simulink model "boostObserver_original"  (R2020a)
settings: Solver=ode45  StartTime=0.0  StopTime=1  FixedStep=0.0005  AbsTol=1e-06  EnableMultiTasking=on
InitFcn:
  | kp=0.01;
  | ki=0.01;
  | 
  | k=2;
  | em=100000000;
  | GE=1/em;
  | GU=k*ki/GE;
  | GCE=k*kp/GU;
model workspace (MAT data in the model file):
  time = 0.8
values from neighbouring files (symbols this model uses):
  A1 = obj.boostConverter.A1    [BoostController.m]    (also in BoostConverter.m = [-obj.R/obj.L 0;0 -1/(obj.Ro*obj.C)]; BuckBoostConverter.m = [-obj.R/obj.L 0;0 -1/(obj.Ro*obj.C)]; obsmc.m = Asigma{1,1}; workspace_atual.mat = [-16.4  0; 0  -3.50877192982])
  A1aug = [-16.4  0  0; 0  -3.50877192982  0; 0  1  0]    [workspace_atual.mat]    (also in workspace_certo.mat)
  A2 = obj.boostConverter.A2    [BoostController.m]    (also in BoostConverter.m = [-obj.R/obj.L -1/obj.L;1/obj.C -1/(obj.Ro*obj.C)]; BuckBoostConverter.m = [-obj.R/obj.L 1/obj.L;-1/obj.C -1/(obj.Ro*obj.C)]; obsmc.m = Asigma{1,2}; workspace_atual.mat = [-16.4  -200; 350.877192982  -3.50877192982])
  B1 = obj.boostConverter.B1    [BoostController.m]    (also in BoostConverter.m = [1/obj.L;0]; BuckBoostConverter.m = [1/obj.L;0]; obsmc.m = Bsigma{1,1}; workspace_atual.mat = [200 0])
  B2aug = [200 0 -2]    [workspace_atual.mat]    (also in workspace_certo.mat)
  c = 0.00285    [workspace_atual.mat]    (also in workspace_certo.mat)
  CiL = [0 1]    [workspace_atual.mat]    (also in workspace_certo.mat)
  Cmatrix = [1  0; 0  1]    [workspace_atual.mat]    (also in workspace_certo.mat)
  CVc = [1 0]    [workspace_atual.mat]    (also in workspace_certo.mat)
  deltaA = [0  200  0; -350.877192982  0  0; 0  0  0]    [workspace_atual.mat]    (also in workspace_certo.mat)
  FaultClass = 0    [BoostFaultSimulation.m]    (also in workspace_atual.mat = 1; workspace_certo.mat = 1)
  ie = equilibriumcurrent(obj,ve)    [BoostConverter.m]    (also in BoostFaultSimulation.m = 7.6251; BuckBoostConverter.m = i_e(obj,ve); workspace_atual.mat = 7.6251; workspace_certo.mat = 7.6251)
  iLFaultSwitch = 0    [BoostFaultSimulation.m]    (also in workspace_atual.mat; workspace_certo.mat)
  iLFaultTime = 1.70    (= 1.7)    [BoostFaultSimulation.m]    (also in workspace_atual.mat; workspace_certo.mat)
  Kg = [-8 -0.8 -2.3]    [workspace_atual.mat]    (also in workspace_certo.mat)
  Lnew1 = [0.000426144297292  -1.37628182296; -0.636691353583  10000.3869597]    [workspace_atual.mat]    (also in workspace_certo.mat = [0.00144628510103  0.00148492117427; 0.000288596381821  0.00)
  Lnew2 = [0.000454345330516  -0.588943865675; 0.999552025739  4999.94512306]    [workspace_atual.mat]    (also in workspace_certo.mat = [0.00251672143174  0.00251025627081; 6.60131109739e-05  6.53)
  LoadAddFactor = 0.30    (= 0.3)    [BoostFaultSimulation.m]    (also in workspace_atual.mat; workspace_certo.mat)
  LoadRemoveFactor = 0.30    (= 0.3)    [BoostFaultSimulation.m]    (also in workspace_atual.mat; workspace_certo.mat)
  Lobsmc = L    [obsmc.m]    (also in workspace_atual.mat = [-39.840516804 -308.588682873 -0.55787282725]; workspace_certo.mat = [-39.840516804 -308.588682873 -0.55787282725])
  R = 0.1    [boostResults2Latex.m]    (also in workspace_atual.mat = 0.082; workspace_certo.mat = 0.082)
  ReconfigSwitch = 0    [BoostFaultSimulation.m]    (also in workspace_atual.mat; workspace_certo.mat)
  ReconfigTime = 1.707    [BoostFaultSimulation.m]    (also in workspace_atual.mat; workspace_certo.mat)
  Ro = 100    [BoostFaultSimulation.m]    (also in boostResults2Latex.m = 10; workspace_atual.mat; workspace_certo.mat)
  Smep = 80    [workspace_atual.mat]    (also in workspace_certo.mat)
  SmFrequency = 7000    [workspace_atual.mat]    (also in workspace_certo.mat)
  SmiLGain = 8    [workspace_atual.mat]    (also in workspace_certo.mat)
  SmIntegralGain = 2.3    [workspace_atual.mat]    (also in workspace_certo.mat)
  SmVcGain = 0.8    [workspace_atual.mat]    (also in workspace_certo.mat)
  SourceAddFactor = 0.10    (= 0.1)    [BoostFaultSimulation.m]    (also in workspace_atual.mat; workspace_certo.mat)
  SourceAddSwitch = 0    [BoostFaultSimulation.m]    (also in workspace_atual.mat; workspace_certo.mat)
  SourceRemoveFactor = 0.10    (= 0.1)    [BoostFaultSimulation.m]    (also in workspace_atual.mat; workspace_certo.mat)
  T_1 = [1 -13715.5123667]    [workspace_atual.mat]    (also in workspace_certo.mat)
  T_2 = [-0.00750867981628 1]    [workspace_atual.mat]    (also in workspace_certo.mat)
  Ts = 0.0001    [workspace_atual.mat]    (also in workspace_certo.mat)
  ueq = 0.5    [workspace_atual.mat]    (also in workspace_certo.mat)
  VcFaultSwitch = 0    [BoostFaultSimulation.m]    (also in workspace_atual.mat; workspace_certo.mat)
  VcFaultTime = 1.70    (= 1.7)    [BoostFaultSimulation.m]    (also in workspace_atual.mat; workspace_certo.mat)
  ve = 380    [BoostFaultSimulation.m]    (also in boostResults2Latex.m = 100; workspace_atual.mat; workspace_certo.mat)
  Wobsmc = W    [obsmc.m]    (also in workspace_atual.mat = [3.6619016063  2.99523180353  1.23384935718; 2.99523180353  ; workspace_certo.mat = [3.66188539077  2.99521892267  1.23384557868; 2.99521892267 )
  x_e = [ie;ve]    [BoostConverter.m]    (also in BuckBoostConverter.m)
  xe = obj.boostConverter.equilibriumstate(ve)    [BoostController.m]    (also in workspace_atual.mat = [7.62509288104 380]; workspace_certo.mat = [7.62509288104 380])
libraries: PhdLibrary x17, neural x12, powerlib_meascontrol x3, dspstat3 x1, powerlib x1
(part 1 of 2)
settings Model: SimulationMode=accelerator  Creator=d13go  LastModifiedBy=d13go
settings SolverCC: MaxConsecutiveZCs=10000  ZeroCrossAlgorithm=Adaptive  DecoupledContinuousIntegration=on  MinimalZcImpactIntegration=on
settings DataIOCC: SaveFinalState=on  SaveState=on  LoggingToFile=on
settings OptimizationCC: DefaultParameterBehavior=Inlined  UseDivisionForNetSlopeComputation=on  GainParamInheritBuiltInType=on  UseFloatMulNetSlope=on  InlineInvariantSignals=on  EfficientFloat2IntCast=on  LifeSpan=1
settings DebuggingCC: ReadBeforeWriteMsg=DisableAll  WriteAfterWriteMsg=DisableAll  WriteAfterReadMsg=DisableAll  AlgebraicLoopMsg=error  MaxConsecutiveZCsMsg=warning  MaskedZcDiagnostic=none  IgnoredZcDiagnostic=none  MultiTaskDSMMsg=none  SFUnexpectedBacktrackingDiag=warning  SFNoUnconditionalDefaultTransitionDiag=warning  ArithmeticOperatorsInVariantConditions=warning
settings HardwareCC: ProdLongLongMode=on
settings ModelReferenceCC: UpdateModelReferenceTargets=IfOutOfDate
settings SFSimCC: SFSimEcho=off  SimUseLocalCustomCode=off  MATLABDynamicMemAlloc=off  CustomCodeUndefinedFunction=UseInterfaceOnly
settings RTWCC: GenerateReport=on  RTWUseLocalCustomCode=off  LaunchReport=on
settings CodeAppCC: ForceParamTrailComments=on
settings GRTTargetCC: TargetLangStandard=C89/C90 (ANSI)  CombineSignalStateStructs=on  MatFileLogging=off  SupportVariableSizeSignals=on
settings ConfigComp: CovMetricSettings=dw  CovHtmlReporting=on  CovSaveCumulativeToWorkspaceVar=on  CovSaveSingleToWorkspaceVar=on  CovExternalEMLEnable=off
settings SimscapeCC: SimscapeNormalizeSystem=off

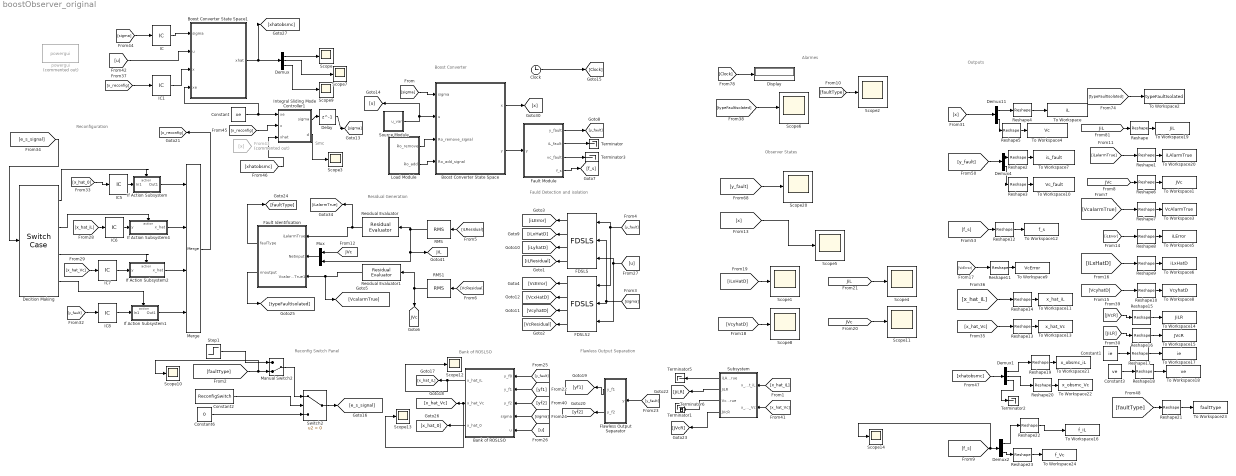
== system boostObserver_original ==
  note: Alarmes
  note: Smc
  note: Fauld Detection and isolation
  note: Outputs
  note: Bank of ROSLSO
  note: Flawless Output
      | Separation
  note: Observer States
  note: Residual Generation
  note: Reconfiguration
  note: Reconfig Switch Panel
  note: Boost Converter
  Bank of ROSLSO : Subsystem
  Boost Converter State Space : Subsystem  AncestorBlock="PhdLibrary/Boost Converter  State Space"  mask(Boots State-Space model){A1=A1, A2=A2, B1=B1, R=R, Ro=Ro, Cmatrix=Cmatrix, c=c, LoadAddFactor=LoadAddFactor, LoadRemoveFactor=LoadRemoveFactor}
      mask prompts: A1 "A1 matrix:"; A2 "A2 matrix:"; B1 "B matrix:"; R "Resistance:"; Ro "Output Resistance:"; Cmatrix "Output Matrix:"; c "Capacitance:"; LoadAddFactor "Load add factor:"; LoadRemoveFactor "Load remove factor"
      mask help: Boots State-Space model
      mask Display: disp('Boost')
  Boost Converter State Space1 : Subsystem  mask(Boots State-Space model){A1=A1, A2=A2, B1=B1, R=R, Ro=Ro, Cmatrix=Cmatrix, c=c, LoadAddFactor=LoadAddFactor, LoadRemoveFactor=LoadRemoveFactor}
      mask prompts: A1 "A1 matrix:"; A2 "A2 matrix:"; B1 "B matrix:"; R "Resistance:"; Ro "Output Resistance:"; Cmatrix "Output Matrix:"; c "Capacitance:"; LoadAddFactor "Load add factor:"; LoadRemoveFactor "Load remove factor"
      mask help: Boots State-Space model
      mask Display: disp('Boost')
  Clock : Clock
  Constant : Constant  Value=xe  VectorParams1D=off
  Constant1 : Constant  Value=ie  VectorParams1D=off
  Constant2 : Constant  Value=ReconfigSwitch
  Constant3 : Constant  Value=ve  VectorParams1D=off
  Constant6 : Constant  Value=0
  Decition Making : SwitchCase  CaseConditions={[0],[1],[2]}
  Delay : Delay  DelayLength=1
  Demux : Demux  Outputs=3
  Demux1 : Demux  Outputs=3
  Demux11 : Demux  Outputs=2
  Demux2 : Demux  Outputs=2
  Demux4 : Demux  Outputs=2
  Display : Display
  FDSLS : PhdLibrary/FDSLS  A1=A1  A2=A2  B1=B1  B2=B2  L=Lnew1  yhat0=[0;0]  x0=[0;0]  Qr=[1 0]
      settings: SourceProductName=Phd Diego
  FDSLS2 : PhdLibrary/FDSLS  A1=A1  A2=A2  B1=B1  B2=B2  L=Lnew2  yhat0=[0;0]  x0=[0;0]  Qr=[0 1]
      settings: SourceProductName=Phd Diego
  Fault Identification : Subsystem
  Fault Module : Subsystem
  Flawless Output Separator : Subsystem  mask(Flawless Output Separator){Cf1=CiL, Cf2=CVc}
      mask prompts: Cf1 "Fault matrix 1"; Cf2 "Fault matrix 2"
      mask help: Separates the 2x1 output
  From43 : From  Commented=on  GotoTag=x
  IC : InitialCondition
  IC{1,5..8} (5 alike) : InitialCondition  Value=[0;0]
  If Action Subsystem : Subsystem  TreatAsAtomicUnit=on
  If Action Subsystem1 : Subsystem  TreatAsAtomicUnit=on
  If Action Subsystem2 : Subsystem  TreatAsAtomicUnit=on
  If Action Subsystem4 : Subsystem  TreatAsAtomicUnit=on
  Integral Sliding Mode Controller1 : Subsystem  mask(Sliding mode controller){KiVc=SmIntegralGain, KVc=SmVcGain, ueq=ueq, Smep=Smep, KiL=SmiLGain, Freq=SmFrequency, x0=[0;0], Ts=0}
      mask prompts: KiVc "Integral voltage gain"; KVc "Voltage gain"; ueq "Equilibrium signal"; Smep "Surface limit layer"; KiL "Current gain"; Freq "Frequency"; x0 "Initial state:"; Ts "Sample Time"
      mask help: Sliding mode controller with integral for boost converter
  Load Module : Subsystem
  Manual Switch2 : ManualSwitch  CurrentSetting=0
  Merge : Merge  Inputs=4
  Mux : Mux  Inputs=2
  RMS : powerlib_meascontrol/Measurements/RMS  TrueRMS=on  Freq=RMSfrequency  RMSInit=0  Ts=Ts
  RMS1 : powerlib_meascontrol/Measurements/RMS  TrueRMS=on  Freq=RMSfrequency  RMSInit=0  Ts=Ts
  Reshape{,1..23} (24 alike) : Reshape
  Residual Evaluator : PhdLibrary/Residual Evaluator  Jth=iLJth
      settings: SourceProductName=Phd Diego
  Residual Evaluator1 : PhdLibrary/Residual Evaluator  Jth=VcJth
      settings: SourceProductName=Phd Diego
  Scope{,1..14,20} (16 alike) : Scope
  Source Module : Subsystem
  Step1 : Step  Time=ReconfigTime  After=FaultClass  SampleTime=0
  Subsystem : Subsystem
  Switch2 : Switch  Criteria=u2 > Threshold
  Terminator{,1..3,5..6} (6 alike) : Terminator
  To Workspace : ToWorkspace  VariableName=iL  SaveFormat=Timeseries  SampleTime=-1
  To Workspace1 : ToWorkspace  VariableName=JVc  SaveFormat=Timeseries  SampleTime=-1
  To Workspace10 : ToWorkspace  VariableName=Vc_fault  SaveFormat=Timeseries  SampleTime=-1
  To Workspace11 : ToWorkspace  VariableName=x_hat_iL  SaveFormat=Timeseries  SampleTime=-1
  To Workspace12 : ToWorkspace  VariableName=f_s  SaveFormat=Timeseries  SampleTime=-1
  To Workspace13 : ToWorkspace  VariableName=x_hat_Vc  SaveFormat=Timeseries  SampleTime=-1
  To Workspace14 : ToWorkspace  VariableName=JiLR  SaveFormat=Timeseries  SampleTime=-1
  To Workspace15 : ToWorkspace  VariableName=JVcR  SaveFormat=Timeseries  SampleTime=-1
  To Workspace16 : ToWorkspace  VariableName=f_iL  SaveFormat=Timeseries  SampleTime=-1
  To Workspace17 : ToWorkspace  VariableName=ie  SaveFormat=Timeseries  SampleTime=-1
  To Workspace18 : ToWorkspace  VariableName=ve  SaveFormat=Timeseries  SampleTime=-1
  To Workspace19 : ToWorkspace  VariableName=JiL  SaveFormat=Timeseries  SampleTime=-1
  To Workspace2 : ToWorkspace  VariableName=typeFaultIsolated  SaveFormat=Timeseries  SampleTime=-1
  To Workspace20 : ToWorkspace  VariableName=iLAlarmTrue  SaveFormat=Timeseries  SampleTime=-1
  To Workspace21 : ToWorkspace  VariableName=x_obsmc_iL  SaveFormat=Timeseries  SampleTime=-1
  To Workspace22 : ToWorkspace  VariableName=x_obsmc_Vc  SaveFormat=Timeseries  SampleTime=-1
  To Workspace23 : ToWorkspace  VariableName=faultType  SaveFormat=Timeseries  SampleTime=-1
  To Workspace24 : ToWorkspace  VariableName=f_Vc  SaveFormat=Timeseries  SampleTime=-1
  To Workspace3 : ToWorkspace  VariableName=VcAlarmTrue  SaveFormat=Timeseries  SampleTime=-1
  To Workspace4 : ToWorkspace  VariableName=Vc  SaveFormat=Timeseries  SampleTime=-1
  To Workspace5 : ToWorkspace  VariableName=iLError  SaveFormat=Timeseries  SampleTime=-1
  To Workspace6 : ToWorkspace  VariableName=iLxHatD  SaveFormat=Timeseries  SampleTime=-1
  To Workspace7 : ToWorkspace  VariableName=iL_fault  SaveFormat=Timeseries  SampleTime=-1
  To Workspace8 : ToWorkspace  VariableName=VcyhatD  SaveFormat=Timeseries  SampleTime=-1
  To Workspace9 : ToWorkspace  VariableName=VcError  SaveFormat=Timeseries  SampleTime=-1
  powergui : powerlib/powergui  Priority=1  Commented=on  SimulationMode=Discrete  SampleTime=50e-6  frequency=60  Iterations=50  frequencyindice=0  Pbase=100e6  ErrMax=1e-4  UnitsV=kV  UnitsW=MW  buscounter=0  FunctionMessages=off  echomessages=off  EnableUseOfTLC=off  CurrentSourceSwitches=off  DisableSnubberDevices=off  DisableRonSwitches=off  DisableVfSwitches=off  DisplayEquations=off  AutomaticDiscreteSolvers=off  SolverType=Tustin/Backward Euler (TBE)  Interpol=off  ExternalGateDelay=off  methode=off  Ts=100  x0status=blocks  SPID=on  SwTol=0  HookPort=off  NonlinearTolerance=1e-4  nMaxIteration=100  ContinueOnMaxIteration=off  RestoreLinks=warning  ResistiveCurrentMeasurement=off  Frange=[0:2:500]  Ylog=off  Xlog=on  ShowGrid=off  save=off  variable=ZData  structure=0  ZoomFFT=off  StartTime=0.0  cycles=1  DisplayStyle=1  fundamental=60  FreqAxis=off  MaxFrequency=1000  frequencyindicesteady=1  RmsSteady=1  display=off
  tag scope: JVc=global, JiL=global
  wires:
  Switch2/1 -> [e_s_signal]
  Reshape9/1 -> To Workspace6/1
  [y_fault] -> FDSLS2/1, FDSLS/1
  Demux4/1 -> Reshape2/1
  If Action Subsystem2/1(x_hat) -> Merge/3
  Decition Making/4 -> If Action Subsystem1/Action
  [iLResidual] -> RMS/1
  [faultType] -> Scope2/1
  [faultType] -> Scope10/1, Manual Switch2/2
  Merge/1 -> [x_reconfig]
  Clock/1 -> [Clock]
  Boost Converter State Space/1(x) -> [x]
  IC7/1 -> If Action Subsystem2/1(y)
  Fault Module/2(iL_fault) -> Terminator/1
  [JVc] -> Scope11/1
  [x_hat_Vc] -> Reshape13/1
  Demux4/2 -> Reshape3/1
  IC5/1 -> If Action Subsystem/1(In1)
  If Action Subsystem1/1(Out1) -> Merge/4
  Manual Switch2/1 -> Switch2/1
  Reshape7/1 -> To Workspace3/1
  Flawless Output Separator/2(y_f2) -> [yf2]
  Load Module/1(Ro_remove) -> Boost Converter State Space/3(Ro_remove_signal)
  [u] -> Bank of ROSLSO/5(u)
  Reshape12/1 -> To Workspace12/1
  [y_fault] -> Flawless Output Separator/1(y)
  Constant6/1 -> Switch2/3
  Reshape2/1 -> To Workspace7/1
  Fault Identification/2(nnoutput) -> [typeFaultIsolated]
  Residual Evaluator/1 -> Fault Identification/1(iLalarmTrue), [iLalarmTrue]
  Mux/1 -> Fault Identification/2(Netinput)
  Decition Making/3 -> If Action Subsystem2/Action
  Decition Making/2 -> If Action Subsystem4/Action
  [JVcR] -> Reshape15/1
  Residual Evaluator1/1 -> [VcalarmTrue], Fault Identification/3(VcalarmTrue1)
  Fault Identification/1(faulType) -> [faultType]
  [y_fault] -> Scope20/1
  [JiL] -> Scope4/1
  [VcyhatD] -> Reshape10/1
  [x] -> Demux11/1
  FDSLS2/2 -> [VcxHatD]
  Load Module/2(Ro_add) -> Boost Converter State Space/4(Ro_add_signal)
  Source Module/1(u_var) -> [u], Boost Converter State Space/2(u)
  Fault Module/4(f_s) -> [f_s]
  Boost Converter State Space/2(y) -> Fault Module/1(y)
  [VcResidual] -> RMS1/1
  [sigma] -> FDSLS2/2, FDSLS/2
  Reshape16/1 -> To Workspace15/1
  Demux11/1 -> Reshape4/1
  Bank of ROSLSO/1(x_hat_iL) -> Scope12/1, [x_hat_iL]
  Reshape13/1 -> To Workspace13/1
  RMS1/1 -> Residual Evaluator1/1, [JVc]
  RMS/1 -> [JiL], Mux/2, Residual Evaluator/1
  Reshape15/1 -> To Workspace14/1
  [iLalarmTrue] -> Reshape1/1
  Reshape1/1 -> To Workspace20/1
  Flawless Output Separator/1(y_f1) -> [yf1]
  Reshape14/1 -> To Workspace11/1
  [sigma] -> Boost Converter State Space/1(sigma)
  [VcError] -> Reshape11/1
  [x] -> Scope5/1
  FDSLS/4 -> [iLResidual]
  FDSLS2/3 -> [VcyhatD]
  [y_fault] -> Bank of ROSLSO/1(y_f0)
  Reshape4/1 -> To Workspace/1
  FDSLS2/1 -> [VcError]
  [VcyhatD] -> Scope8/1
  Reshape11/1 -> To Workspace9/1
  [y_fault] -> Demux4/1
  FDSLS/3 -> [iLyhatD]
  Fault Module/3(vc_fault) -> Terminator3/1
  Reshape8/1 -> To Workspace5/1
  Demux11/2 -> Reshape5/1
  [f_s] -> Reshape12/1
  [x_hat_iL] -> Reshape14/1
  FDSLS/1 -> [iLError]
  Step1/1 -> Manual Switch2/1
  If Action Subsystem/1(Out1) -> Merge/1
  [typeFaultIsolated] -> To Workspace2/1
  [u] -> FDSLS2/3, FDSLS/3
  [iLError] -> Reshape8/1
  FDSLS2/4 -> [VcResidual]
  If Action Subsystem4/1(x_hat) -> Merge/2
  [x_hat_0] -> IC5/1
  Reshape6/1 -> To Workspace1/1
  [y_fault] -> IC8/1
  Fault Module/1(y_fault) -> [y_fault]
  [x_hat_Vc] -> IC7/1
  [typeFaultIsolated] -> Scope6/1
  [VcalarmTrue] -> Reshape7/1
  [iLxHatD] -> Reshape9/1
  Reshape3/1 -> To Workspace10/1
  IC8/1 -> If Action Subsystem1/1(In1)
  IC6/1 -> If Action Subsystem4/1(y)
  [x_hat_iL] -> IC6/1
  [JiL] -> Reshape/1
  [e_s_signal] -> Decition Making/1
  [sigma] -> Bank of ROSLSO/4(sigma)
  [JVc] -> Reshape6/1
  Reshape/1 -> To Workspace19/1
  Reshape5/1 -> To Workspace4/1
  [Clock] -> Display/1
  Reshape10/1 -> To Workspace8/1
  Decition Making/1 -> If Action Subsystem/Action
  [iLxHatD] -> Scope1/1
  FDSLS/2 -> [iLxHatD]
  [JiLR] -> Reshape16/1
  Constant2/1 -> Switch2/2
  [JVc] -> Mux/1
  Subsystem/1(iLAlarmTrue) -> Terminator5/1
  Subsystem/2(JiLR) -> [JiLR]
  Subsystem/3(VcAlarmTrue) -> Terminator6/1
  Subsystem/4(JVcR) -> [JVcR]
  [x_hat_iL] -> Subsystem/1(x_hat_iL)
  [yf1] -> Bank of ROSLSO/2(y_f1)
  [yf2] -> Bank of ROSLSO/3(y_f2)
  Bank of ROSLSO/3(x_hat_0) -> [x_hat_0]
  [x_hat_Vc] -> Subsystem/2(x_hat_Vc)
  Integral Sliding Mode Controller1/2(d) -> Scope3/1
  Constant/1 -> Integral Sliding Mode Controller1/1(xe), Boost Converter State Space1/4(xe)
  Demux/2 -> Scope7/1
  Boost Converter State Space1/1(xhat) -> [xhatobsmc], Demux/1
  Demux/3 -> Scope9/1
  [sigma] -> IC/1
  Demux/1 -> Scope/1
  [u] -> Boost Converter State Space1/2(u)
  IC/1 -> Boost Converter State Space1/1(sigma)
  IC1/1 -> Boost Converter State Space1/3(x)
  [x_reconfig] -> Integral Sliding Mode Controller1/2(x)
  [x_reconfig] -> IC1/1
  Bank of ROSLSO/2(x_hat_Vc) -> Scope13/1, [x_hat_Vc]
  [xhatobsmc] -> Integral Sliding Mode Controller1/3(xhat)
  Integral Sliding Mode Controller1/1(sigma) -> Delay/1
  Delay/1 -> [sigma]
  Constant1/1 -> Reshape17/1
  Reshape17/1 -> To Workspace17/1
  Constant3/1 -> Reshape18/1
  Reshape18/1 -> To Workspace18/1
  [xhatobsmc] -> Demux1/1
  Reshape19/1 -> To Workspace21/1
  Demux1/1 -> Reshape19/1
  Reshape20/1 -> To Workspace22/1
  Demux1/2 -> Reshape20/1
  Demux1/3 -> Terminator2/1
  [faultType] -> Reshape21/1
  Reshape21/1 -> To Workspace23/1
  Reshape22/1 -> To Workspace16/1
  Demux2/1 -> Reshape22/1
  Reshape23/1 -> To Workspace24/1
  Demux2/2 -> Reshape23/1
  [f_s] -> Scope14/1, Demux2/1

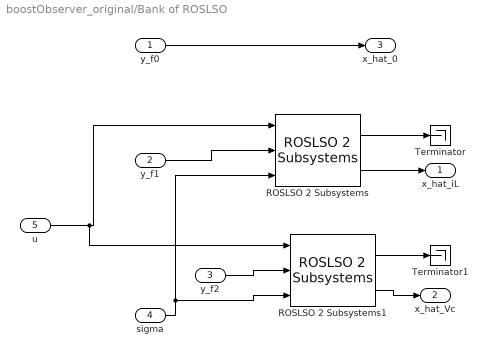
== system boostObserver_original/Bank of ROSLSO ==
  y_f0 : Inport
  y_f1 : Inport  Port=2
  y_f2 : Inport  Port=3
  sigma : Inport  Port=4
  u : Inport  Port=5
  ROSLSO 2 Subsystems : PhdLibrary/ROSLSO  2 Subsystems  B1=B1f  B2=B2f  T=T_1  F1=F_11  F2=F_12  L1=L_11  L2=L_12  Q=Q_1  z0=0
      settings: SourceProductName=Phd Diego
  ROSLSO 2 Subsystems1 : PhdLibrary/ROSLSO  2 Subsystems  B1=B1f  B2=B2f  T=T_2  F1=F_21  F2=F_22  L1=L_21  L2=L_22  Q=Q_2  z0=0
      settings: SourceProductName=Phd Diego
  Terminator : Terminator
  Terminator1 : Terminator
  x_hat_iL : Outport
  x_hat_Vc : Outport  Port=2
  x_hat_0 : Outport  Port=3
  wires:
  sigma/1 -> ROSLSO 2 Subsystems/3, ROSLSO 2 Subsystems1/3
  y_f1/1 -> ROSLSO 2 Subsystems/2
  y_f2/1 -> ROSLSO 2 Subsystems1/2
  ROSLSO 2 Subsystems1/2 -> x_hat_Vc/1
  ROSLSO 2 Subsystems/2 -> x_hat_iL/1
  ROSLSO 2 Subsystems/1 -> Terminator/1
  ROSLSO 2 Subsystems1/1 -> Terminator1/1
  y_f0/1 -> x_hat_0/1
  u/1 -> ROSLSO 2 Subsystems1/1, ROSLSO 2 Subsystems/1

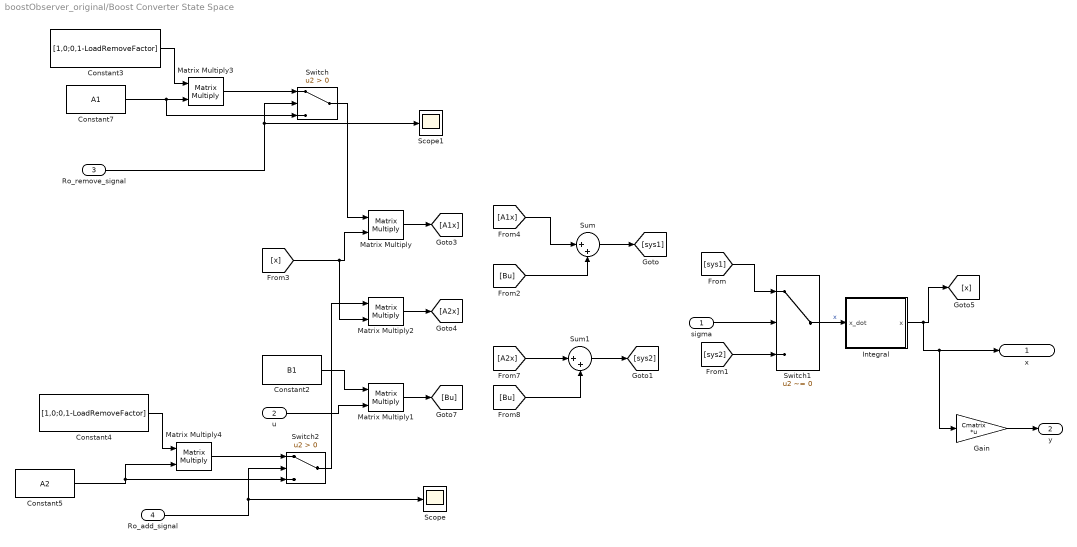
== system boostObserver_original/Boost Converter State Space ==
  sigma : Inport
  u : Inport  Port=2
  Ro_remove_signal : Inport  Port=3
  Ro_add_signal : Inport  Port=4
  Constant2 : Constant  Value=B1  VectorParams1D=off
  Constant3 : Constant  Value=[1,0;0,1-LoadRemoveFactor]  VectorParams1D=off
  Constant4 : Constant  Value=[1,0;0,1-LoadRemoveFactor]  VectorParams1D=off
  Constant5 : Constant  Value=A2  VectorParams1D=off
  Constant7 : Constant  Value=A1  VectorParams1D=off
  Gain : Gain  Gain=Cmatrix  Multiplication=Matrix(K*u)
  Integral : Subsystem
  Matrix Multiply{,1..4} (5 alike) : Product  Multiplication=Matrix(*)
  Scope : Scope
  Scope1 : Scope
  Sum : Sum  Inputs=|++
  Sum1 : Sum  Inputs=|++
  Switch : Switch  Criteria=u2 > Threshold
  Switch1 : Switch  Criteria=u2 ~= 0
  Switch2 : Switch  Criteria=u2 > Threshold
  x : Outport
  y : Outport  Port=2
  wires:
  Switch2/1 -> Matrix Multiply2/1
  Ro_add_signal/1 -> Scope/1, Switch2/2
  Constant5/1 -> Matrix Multiply4/2, Switch2/3
  Matrix Multiply4/1 -> Switch2/1
  Constant4/1 -> Matrix Multiply4/1
  Switch/1 -> Matrix Multiply/1
  Ro_remove_signal/1 -> Scope1/1, Switch/2
  Matrix Multiply3/1 -> Switch/1
  Constant7/1 -> Switch/3, Matrix Multiply3/2
  Constant3/1 -> Matrix Multiply3/1
  Gain/1 -> y/1
  Integral/1(x) -> [x], x/1, Gain/1
  u/1 -> Matrix Multiply1/2
  Matrix Multiply1/1 -> [Bu]
  Constant2/1 -> Matrix Multiply1/1
  sigma/1 -> Switch1/2
  [A2x] -> Sum1/1
  Switch1/1 -> Integral/1(x_dot)  "x"
  Sum1/1 -> [sys2]
  Sum/1 -> [sys1]
  Matrix Multiply/1 -> [A1x]
  Matrix Multiply2/1 -> [A2x]
  [Bu] -> Sum/2
  [Bu] -> Sum1/2
  [x] -> Matrix Multiply/2, Matrix Multiply2/2
  [A1x] -> Sum/1
  [sys1] -> Switch1/1
  [sys2] -> Switch1/3

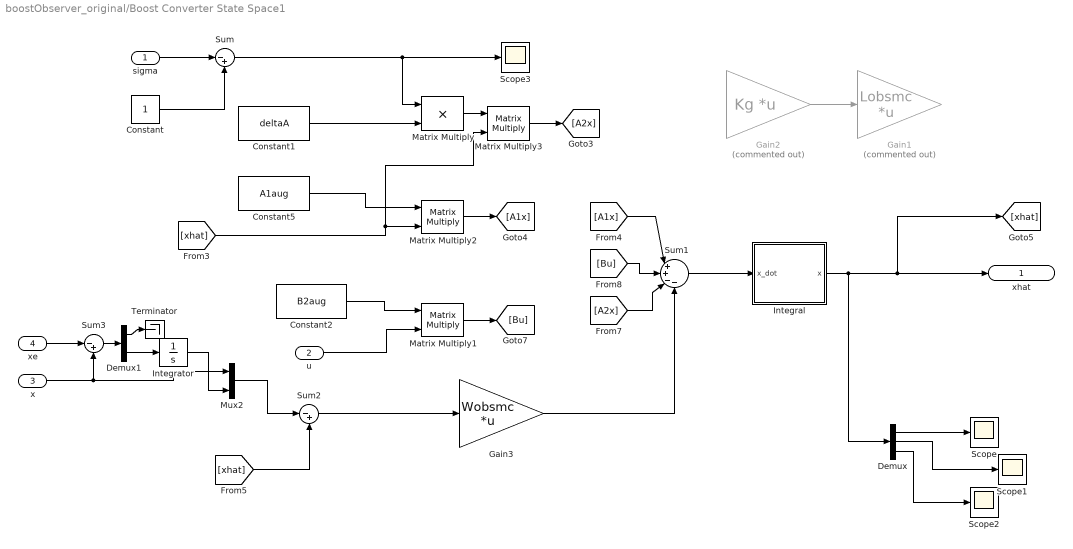
== system boostObserver_original/Boost Converter State Space1 ==
  sigma : Inport
  u : Inport  Port=2
  x : Inport  Port=3
  xe : Inport  Port=4
  Constant : Constant
  Constant1 : Constant  Value=deltaA  VectorParams1D=off
  Constant2 : Constant  Value=B2aug  VectorParams1D=off
  Constant5 : Constant  Value=A1aug  VectorParams1D=off
  Demux : Demux  Outputs=3
  Demux1 : Demux  Outputs=2
  Gain1 : Gain  Commented=on  Gain=Lobsmc  Multiplication=Matrix(K*u)
  Gain2 : Gain  Commented=on  Gain=Kg  Multiplication=Matrix(K*u)
  Gain3 : Gain  Gain=Wobsmc  Multiplication=Matrix(K*u)
  Integral : Subsystem
  Integrator : Integrator
  Matrix Multiply : Product
  Matrix Multiply1 : Product  Multiplication=Matrix(*)
  Matrix Multiply2 : Product  Multiplication=Matrix(*)
  Matrix Multiply3 : Product  Multiplication=Matrix(*)
  Mux2 : Mux  Inputs=2
  Scope{,1..3} (4 alike) : Scope
  Sum : Sum  Inputs=|-+
  Sum1 : Sum  Inputs=|++--
  Sum2 : Sum  Inputs=|-+
  Sum3 : Sum  Inputs=|-+
  Terminator : Terminator
  xhat : Outport
  wires:
  u/1 -> Matrix Multiply1/2
  Matrix Multiply1/1 -> [Bu]
  Constant2/1 -> Matrix Multiply1/1
  Matrix Multiply2/1 -> [A1x]
  [Bu] -> Sum1/2
  [xhat] -> Matrix Multiply3/2, Matrix Multiply2/2
  [xhat] -> Sum2/2
  Demux/2 -> Scope1/1
  Integral/1(x) -> [xhat], xhat/1, Demux/1
  Demux/1 -> Scope/1
  Demux/3 -> Scope2/1
  Gain2/1 -> Gain1/1
  Constant5/1 -> Matrix Multiply2/1
  Sum1/1 -> Integral/1(x_dot)
  Constant1/1 -> Matrix Multiply/2
  Matrix Multiply/1 -> Matrix Multiply3/1
  Matrix Multiply3/1 -> [A2x]
  sigma/1 -> Sum/1
  Sum/1 -> Scope3/1, Matrix Multiply/1
  Constant/1 -> Sum/2
  Sum2/1 -> Gain3/1
  xe/1 -> Sum3/1
  x/1 -> Mux2/1, Sum3/2
  Sum3/1 -> Demux1/1
  Demux1/2 -> Integrator/1
  Integrator/1 -> Mux2/2
  Demux1/1 -> Terminator/1
  Mux2/1 -> Sum2/1
  [A1x] -> Sum1/1
  [A2x] -> Sum1/3
  Gain3/1 -> Sum1/4

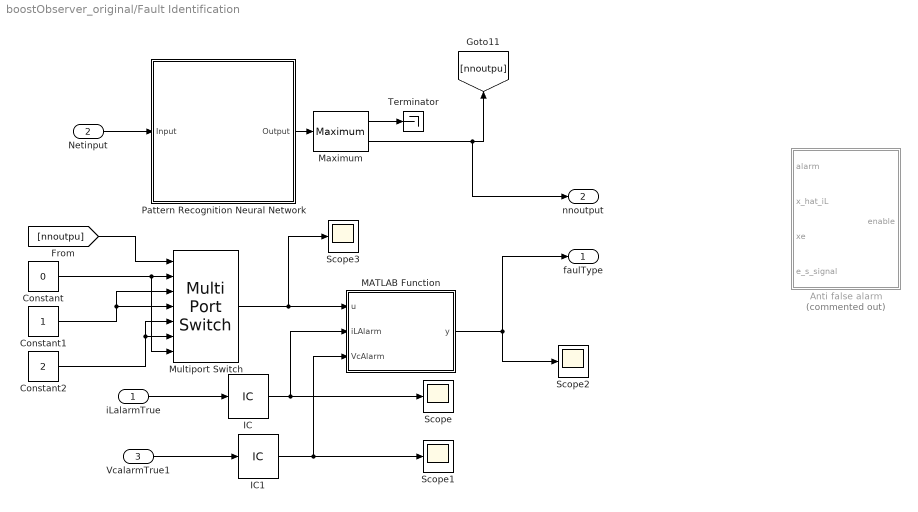
== system boostObserver_original/Fault Identification ==
  iLalarmTrue : Inport
  Netinput : Inport  Port=2
  VcalarmTrue1 : Inport  Port=3
  Anti false alarm : Subsystem  Commented=on
  Constant : Constant  Value=0
  Constant1 : Constant
  Constant2 : Constant  Value=2
  IC : InitialCondition  Value=0
  IC1 : InitialCondition  Value=0
  MATLAB Function : MATLAB Function  TreatAsAtomicUnit=on
  Maximum : dspstat3/Maximum  operation=maximum  fcn=Value and Index  indexBase=One  operateOver=Each column  Dimension=1  InputProcessing=Columns as channels (frame based)  reset=None  roiEnable=off  roiType=Rectangles  roiPortion=Entire ROI  roiOutput=Individual statistics for each ROI  roiFlag=off  roundingMode=Floor  overflowMode=off  accumDataTypeStr=Inherit: Same as product output  accumLastDataTypeStr=Inherit: Same as product output
  Multiport Switch : MultiPortSwitch  Inputs=5  DataPortForDefault=Additional data port
  Pattern Recognition Neural Network : Subsystem
      mask help: Pattern Recognition Neural Network
      mask Display: e = 0.06;c1 = [120 150 230]/255;c2 = ([120 150 230]+0)/383;c3 = ([120 150 230]+128)/383;patch([0 1 1 0],[0 0 1 1],c1);patch([0 1 1 1-e 1-e 0+e],[0 0 1 1-e 0+e 0+e],c2);patch([0 0 1 1-e 0+e 0+e],[0 1 1 1-e 1-e 0+e],c3);plot([0 1 1 0 0],[0 0 1 1 0]);fprintf('NNET');port_label('input',1,' Input');port_label('output',1,'Output ');
  Scope{,1..3} (4 alike) : Scope
  Terminator : Terminator
  faulType : Outport
  nnoutput : Outport  Port=2
  wires:
  Maximum/1 -> Terminator/1
  Pattern Recognition Neural Network/1(Output) -> Maximum/1
  Maximum/2 -> nnoutput/1, [nnoutpu]
  Constant/1 -> Multiport Switch/7, Multiport Switch/2
  Constant1/1 -> Multiport Switch/4, Multiport Switch/3
  Constant2/1 -> Multiport Switch/6, Multiport Switch/5
  Netinput/1 -> Pattern Recognition Neural Network/1(Input)
  [nnoutpu] -> Multiport Switch/1
  VcalarmTrue1/1 -> IC1/1
  Multiport Switch/1 -> Scope3/1, MATLAB Function/1(u)
  iLalarmTrue/1 -> IC/1
  IC/1 -> MATLAB Function/2(iLAlarm), Scope/1
  IC1/1 -> MATLAB Function/3(VcAlarm), Scope1/1
  MATLAB Function/1(y) -> Scope2/1, faulType/1

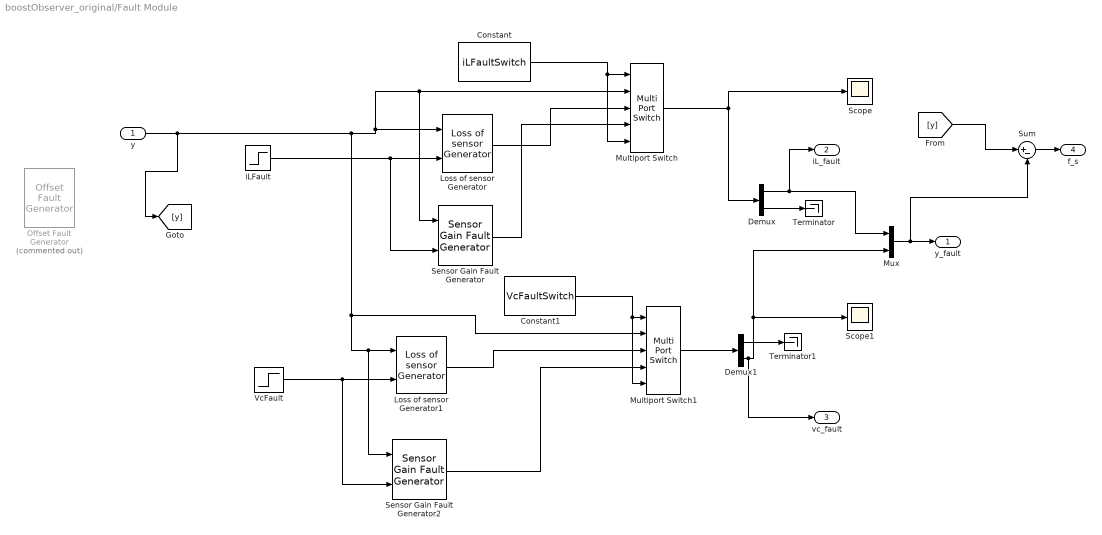
== system boostObserver_original/Fault Module ==
  y : Inport
  Constant : Constant  Value=iLFaultSwitch
  Constant1 : Constant  Value=VcFaultSwitch
  Demux : Demux  Outputs=2
  Demux1 : Demux  Outputs=2
  Loss of sensor Generator : PhdLibrary/Loss of sensor Generator
      settings: SourceProductName=Phd Diego
  Loss of sensor Generator1 : PhdLibrary/Loss of sensor Generator
      settings: SourceProductName=Phd Diego
  Multiport Switch : MultiPortSwitch  DataPortOrder=Zero-based contiguous  DataPortForDefault=Additional data port  zeroidx=on
  Multiport Switch1 : MultiPortSwitch  DataPortOrder=Zero-based contiguous  DataPortForDefault=Additional data port  zeroidx=on
  Mux : Mux  Inputs=2
  Offset Fault Generator : PhdLibrary/Offset Fault Generator  Commented=on  s1gain=20  s2gain=20
      settings: SourceProductName=Phd Diego
  Scope : Scope
  Scope1 : Scope
  Sensor Gain Fault Generator : PhdLibrary/Sensor Gain Fault Generator  s1gain=iLGainFaultFactor  s2gain=VcGainFaultFactor
      settings: SourceProductName=Phd Diego
  Sensor Gain Fault Generator2 : PhdLibrary/Sensor Gain Fault Generator  s1gain=iLGainFaultFactor  s2gain=VcGainFaultFactor
      settings: SourceProductName=Phd Diego
  Sum : Sum  Inputs=|+-
  Terminator : Terminator
  Terminator1 : Terminator
  VcFault : Step  Time=VcFaultTime  After=2  SampleTime=0
  iLFault : Step  Time=iLFaultTime  SampleTime=0
  y_fault : Outport
  iL_fault : Outport  Port=2
  vc_fault : Outport  Port=3
  f_s : Outport  Port=4
  wires:
  iLFault/1 -> Sensor Gain Fault Generator/2, Loss of sensor Generator/2
  y/1 -> [y], Multiport Switch1/2, Sensor Gain Fault Generator2/1, Loss of sensor Generator1/1, Sensor Gain Fault Generator/1, Multiport Switch/2, Loss of sensor Generator/1
  VcFault/1 -> Sensor Gain Fault Generator2/2, Loss of sensor Generator1/2
  Constant/1 -> Multiport Switch/5, Multiport Switch/1
  Constant1/1 -> Multiport Switch1/5, Multiport Switch1/1
  Multiport Switch/1 -> Demux/1, Scope/1
  Multiport Switch1/1 -> Demux1/1
  Demux/2 -> Terminator/1
  Demux/1 -> iL_fault/1, Mux/1
  Mux/1 -> Sum/2, y_fault/1
  Demux1/1 -> Terminator1/1
  Demux1/2 -> vc_fault/1, Mux/2, Scope1/1
  Loss of sensor Generator/1 -> Multiport Switch/3
  Sensor Gain Fault Generator/1 -> Multiport Switch/4
  Sensor Gain Fault Generator2/1 -> Multiport Switch1/4
  Loss of sensor Generator1/1 -> Multiport Switch1/3
  [y] -> Sum/1
  Sum/1 -> f_s/1

== system boostObserver_original/Flawless Output Separator ==
  y : Inport
  Matrizes A1 : Constant  Value=Cf2  VectorParams1D=off
  Matrizes A2 : Constant  Value=Cf1  VectorParams1D=off
  Product : Product  Multiplication=Matrix(*)
  Product1 : Product  Multiplication=Matrix(*)
  y_f1 : Outport
  y_f2 : Outport  Port=2
  wires:
  y/1 -> Product1/2, Product/2
  Matrizes A2/1 -> Product/1
  Matrizes A1/1 -> Product1/1
  Product/1 -> y_f1/1
  Product1/1 -> y_f2/1

== system boostObserver_original/If Action Subsystem ==
  In1 : Inport
  Action Port : ActionPort  ActionPortLabel=case [ 0 ]:
  Out1 : Outport
  wires:
  In1/1 -> Out1/1

== system boostObserver_original/If Action Subsystem1 ==
  In1 : Inport
  Action Port : ActionPort  ActionPortLabel=default:
  Out1 : Outport
  wires:
  In1/1 -> Out1/1

== system boostObserver_original/If Action Subsystem2 ==
  y : Inport
  Action Port : ActionPort  ActionPortLabel=case [ 2 ]:
  x_hat : Outport
  wires:
  y/1 -> x_hat/1

== system boostObserver_original/If Action Subsystem4 ==
  y : Inport
  Action Port : ActionPort  ActionPortLabel=case [ 1 ]:
  x_hat : Outport
  wires:
  y/1 -> x_hat/1

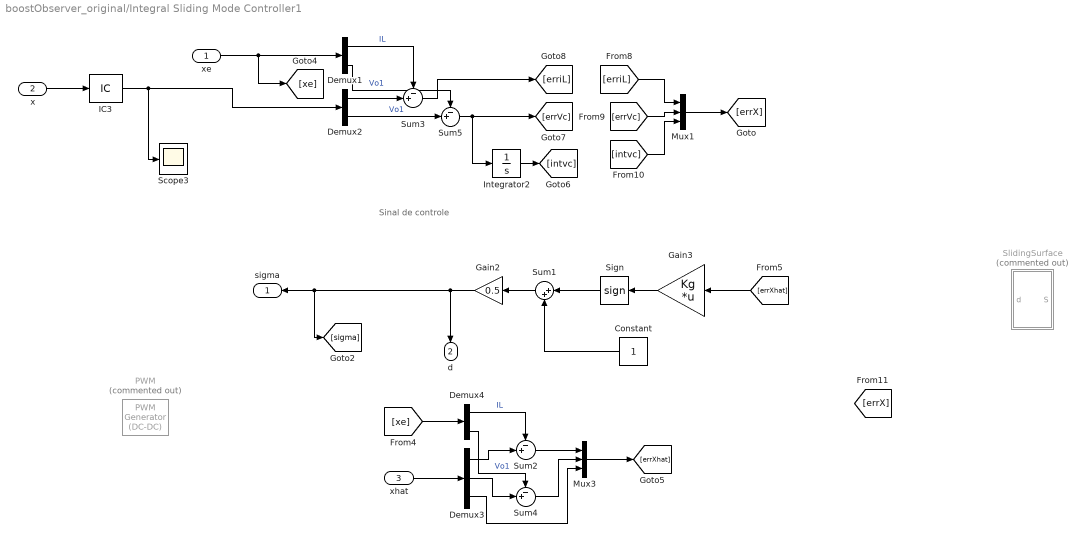
== system boostObserver_original/Integral Sliding Mode Controller1 ==
  note: Sinal de controle
  xe : Inport
  x : Inport  Port=2
  xhat : Inport  Port=3
  Constant : Constant
  Demux1 : Demux  Outputs=2
  Demux2 : Demux  Outputs=2
  Demux3 : Demux  Outputs=3
  Demux4 : Demux  Outputs=2
  Gain2 : Gain  Gain=0.5
  Gain3 : Gain  Gain=Kg  Multiplication=Matrix(K*u)
  IC3 : InitialCondition  Value=x0
  Integrator2 : Integrator
  Mux1 : Mux  Inputs=3
  Mux3 : Mux  Inputs=3
  PWM : powerlib_meascontrol/Pulse & Signal Generators/PWM Generator (DC-DC)  Commented=on  Fsw=Freq  Ts=Ts
  Scope3 : Scope
  Sign : Signum
  SlidingSurface : Subsystem  Commented=on  mask(Sliding mode limit layer){Smep=Smep}
      mask prompts: Smep "Limit layer value"
      mask help: Define a limit layer for the sliding mode signal
      mask DialogControl ParametersGroupVar Prompt: Parameters
  Sum1 : Sum  Inputs=|++
  Sum{2..5} (4 alike) : Sum  Inputs=-+|
  sigma : Outport
  d : Outport  Port=2
  wires:
  IC3/1 -> Scope3/1, Demux2/1
  xe/1 -> [xe], Demux1/1
  x/1 -> IC3/1
  Sum1/1 -> Gain2/1
  Constant/1 -> Sum1/2
  Demux1/2 -> Sum5/1  "Vo1"
  Demux2/2 -> Sum5/2  "Vo1"
  Sum5/1 -> Integrator2/1, [errVc]
  Demux1/1 -> Sum3/1  "IL"
  Demux2/1 -> Sum3/2
  Sum3/1 -> [erriL]
  Integrator2/1 -> [intvc]
  [erriL] -> Mux1/1
  [errVc] -> Mux1/2
  [intvc] -> Mux1/3
  Mux1/1 -> [errX]
  Gain2/1 -> [sigma], sigma/1, d/1
  Demux3/1 -> Sum2/2
  [xe] -> Demux4/1
  Demux4/1 -> Sum2/1  "IL"
  Demux4/2 -> Sum4/1  "Vo1"
  Demux3/2 -> Sum4/2
  Sum2/1 -> Mux3/1
  Mux3/1 -> [errXhat]
  Sum4/1 -> Mux3/2
  Demux3/3 -> Mux3/3
  Gain3/1 -> Sign/1
  Sign/1 -> Sum1/1
  xhat/1 -> Demux3/1
  [errXhat] -> Gain3/1

== system boostObserver_original/Load Module ==
  Load_add_switch : PhdLibrary/Step Perturbation  SignalSwitch=LoadAddSignalSwitch  InitialMagnitude=0  InitialTime=LoadAddTime  Magnitude=1  Duration=LoadAddDuration  enabled=LoadAddSwitch
      settings: SourceProductName=Phd Diego
  Load_remove_switch : PhdLibrary/Step Perturbation  SignalSwitch=LoadRemoveSignalSwitch  InitialMagnitude=0  InitialTime=LoadRemoveTime  Magnitude=1  Duration=LoadRemoveDuration  enabled=LoadRemoveSwitch
      settings: SourceProductName=Phd Diego
  Ro_remove : Outport
  Ro_add : Outport  Port=2
  wires:
  Load_remove_switch/1 -> Ro_remove/1
  Load_add_switch/1 -> Ro_add/1

== system boostObserver_original/Source Module ==
  Constant1 : Constant  Value=SourceAddSwitch  VectorParams1D=off
  Constant11 : Constant  Value=u
  Source_add_switch : PhdLibrary/Step Perturbation  SignalSwitch=SourceAddSignalSwitch  InitialMagnitude=0  InitialTime=SourceAddTime  Magnitude=SourceAddFactor*u  Duration=SourceAddDuration  enabled=SourceAddSwitch
      settings: SourceProductName=Phd Diego
  Source_remove_switch : PhdLibrary/Step Perturbation  SignalSwitch=SourceRemoveSignalSwitch  InitialMagnitude=0  InitialTime=SourceRemoveTime  Magnitude=-SourceRemoveFactor*u  Duration=SourceRemoveDuration  enabled=SourceRemoveSwitch
      settings: SourceProductName=Phd Diego
  Sum : Sum  Inputs=|++
  Sum1 : Sum  Inputs=|++
  Switch : Switch  Criteria=u2 > Threshold
  u_var : Outport
  wires:
  Sum1/1 -> Switch/3
  Sum/1 -> Switch/1
  Constant11/1 -> Sum1/1, Sum/1
  Switch/1 -> u_var/1
  Source_add_switch/1 -> Sum/2
  Source_remove_switch/1 -> Sum1/2
  Constant1/1 -> Switch/2

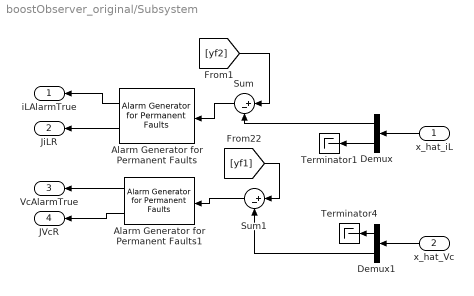
== system boostObserver_original/Subsystem ==
  x_hat_iL : Inport
  x_hat_Vc : Inport  Port=2
  Alarm Generator for Permanent Faults : PhdLibrary/Alarm Generator for Permanent Faults  Jth=0  r0=0
      settings: SourceProductName=Phd Diego
  Alarm Generator for Permanent Faults1 : PhdLibrary/Alarm Generator for Permanent Faults  Jth=0  r0=0
      settings: SourceProductName=Phd Diego
  Demux : Demux  Outputs=2
  Demux1 : Demux  Outputs=2
  Sum : Sum  Inputs=|+-
  Sum1 : Sum  Inputs=|+-
  Terminator1 : Terminator
  Terminator4 : Terminator
  iLAlarmTrue : Outport
  JiLR : Outport  Port=2
  VcAlarmTrue : Outport  Port=3
  JVcR : Outport  Port=4
  wires:
  [yf1] -> Sum1/1
  Alarm Generator for Permanent Faults1/2 -> JVcR/1
  [yf2] -> Sum/1
  Sum1/1 -> Alarm Generator for Permanent Faults1/1
  Sum/1 -> Alarm Generator for Permanent Faults/1
  Alarm Generator for Permanent Faults/2 -> JiLR/1
  Alarm Generator for Permanent Faults/1 -> iLAlarmTrue/1
  Alarm Generator for Permanent Faults1/1 -> VcAlarmTrue/1
  Demux/2 -> Terminator1/1
  Demux/1 -> Sum/2
  x_hat_iL/1 -> Demux/1
  Demux1/1 -> Terminator4/1
  Demux1/2 -> Sum1/2
  x_hat_Vc/1 -> Demux1/1

== system boostObserver_original/Boost Converter State Space/Integral ==
  x_dot : Inport
  Ground : Ground
  Ground1 : Ground
  IC : InitialCondition  Value=[0;0]
  Integrator1 : Integrator  InitialConditionSource=external  InitialCondition=[-x_e; 0; 0]
  Mux : Mux  Inputs=2
  x : Outport
  wires:
  Mux/1 -> IC/1
  Ground/1 -> Mux/1
  Ground1/1 -> Mux/2
  IC/1 -> Integrator1/2
  Integrator1/1 -> x/1
  x_dot/1 -> Integrator1/1

== system boostObserver_original/Boost Converter State Space1/Integral ==
  x_dot : Inport
  Ground : Ground
  Ground1 : Ground
  Ground2 : Ground
  IC : InitialCondition  Value=[0;0;0]
  Integrator1 : Integrator  InitialConditionSource=external  InitialCondition=[-x_e; 0; 0]
  Mux : Mux  Inputs=3
  x : Outport
  wires:
  Mux/1 -> IC/1
  Ground/1 -> Mux/1
  Ground1/1 -> Mux/2
  IC/1 -> Integrator1/2
  Integrator1/1 -> x/1
  x_dot/1 -> Integrator1/1
  Ground2/1 -> Mux/3

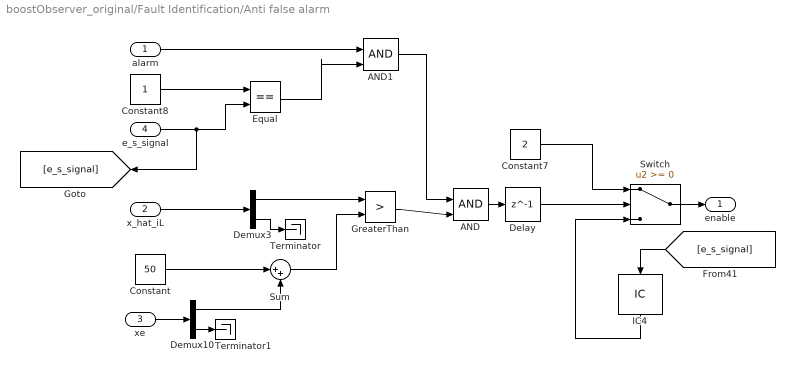
== system boostObserver_original/Fault Identification/Anti false alarm ==
  alarm : Inport
  x_hat_iL : Inport  Port=2
  xe : Inport  Port=3
  e_s_signal : Inport  Port=4
  AND : Logic  IconShape=distinctive  AllPortsSameDT=off  OutDataTypeStr=boolean
  AND1 : Logic  IconShape=distinctive  AllPortsSameDT=off  OutDataTypeStr=boolean
  Constant : Constant  Value=50
  Constant7 : Constant  Value=2
  Constant8 : Constant
  Delay : Delay  DelayLength=1
  Demux10 : Demux  Outputs=2
  Demux3 : Demux  Outputs=2
  Equal : RelationalOperator  Operator===  OutDataTypeStr=boolean  RndMeth=Simplest
  GreaterThan : RelationalOperator  Operator=>  OutDataTypeStr=boolean  RndMeth=Simplest
  IC4 : InitialCondition
  Sum : Sum  Inputs=|++
  Switch : Switch
  Terminator : Terminator
  Terminator1 : Terminator
  enable : Outport
  wires:
  IC4/1 -> Switch/3
  [e_s_signal] -> IC4/1
  AND/1 -> Delay/1
  Constant/1 -> Sum/1
  AND1/1 -> AND/1
  Sum/1 -> GreaterThan/2
  GreaterThan/1 -> AND/2
  Delay/1 -> Switch/2
  Demux3/1 -> GreaterThan/1
  Constant8/1 -> Equal/1
  Equal/1 -> AND1/2
  Demux10/1 -> Sum/2
  Constant7/1 -> Switch/1
  Demux10/2 -> Terminator1/1
  x_hat_iL/1 -> Demux3/1
  Demux3/2 -> Terminator/1
  xe/1 -> Demux10/1
  alarm/1 -> AND1/1
  e_s_signal/1 -> [e_s_signal], Equal/2
  Switch/1 -> enable/1

== system boostObserver_original/Fault Identification/Pattern Recognition Neural Network ==
  Input : Inport  PortDimensions=2
      mask Display: e = 0.06;c1 = [120 230 180]/255;c2 = ([120 230 180]+0)/(256+128);c3 = ([120 230 180]+128)/(256+128);patch([0 1 1 0],[0 0 1 1],c1);patch([0 1 1 1-e 1-e 0+e],[0 0 1 1-e 0+e 0+e],c2);patch([0 0 1 1-e 0+e 0+e],[0 1 1 1-e 1-e 0+e],c3);plot([0 1 1 0 0],[0 0 1 1 0]);
  Layer 1 : Subsystem
      mask Display: e = 0.06;c1 = [120 150 230]/255;c2 = ([120 150 230]+0)/383;c3 = ([120 150 230]+128)/383;patch([0 1 1 0],[0 0 1 1],c1);patch([0 1 1 1-e 1-e 0+e],[0 0 1 1-e 0+e 0+e],c2);patch([0 0 1 1-e 0+e 0+e],[0 1 1 1-e 1-e 0+e],c3);plot([0 1 1 0 0],[0 0 1 1 0]);
  Layer 2 : Subsystem
      mask Display: e = 0.06;c1 = [120 150 230]/255;c2 = ([120 150 230]+0)/383;c3 = ([120 150 230]+128)/383;patch([0 1 1 0],[0 0 1 1],c1);patch([0 1 1 1-e 1-e 0+e],[0 0 1 1-e 0+e 0+e],c2);patch([0 0 1 1-e 0+e 0+e],[0 1 1 1-e 1-e 0+e],c3);plot([0 1 1 0 0],[0 0 1 1 0]);
  Process Input 1 : Subsystem
      mask Display: e = 0.06;c1 = [120 150 230]/255;c2 = ([120 150 230]+0)/383;c3 = ([120 150 230]+128)/383;patch([0 1 1 0],[0 0 1 1],c1);patch([0 1 1 1-e 1-e 0+e],[0 0 1 1-e 0+e 0+e],c2);patch([0 0 1 1-e 0+e 0+e],[0 1 1 1-e 1-e 0+e],c3);plot([0 1 1 0 0],[0 0 1 1 0]);
  Process Output 1 : Subsystem
      mask Display: e = 0.06;c1 = [120 150 230]/255;c2 = ([120 150 230]+0)/383;c3 = ([120 150 230]+128)/383;patch([0 1 1 0],[0 0 1 1],c1);patch([0 1 1 1-e 1-e 0+e],[0 0 1 1-e 0+e 0+e],c2);patch([0 0 1 1-e 0+e 0+e],[0 1 1 1-e 1-e 0+e],c3);plot([0 1 1 0 0],[0 0 1 1 0]);
  Output : Outport  InitialOutput=[0;0;0;0;0]
      mask Display: e = 0.06;c1 = [120 230 180]/255;c2 = ([120 230 180]+0)/(256+128);c3 = ([120 230 180]+128)/(256+128);patch([0 1 1 0],[0 0 1 1],c1);patch([0 1 1 1-e 1-e 0+e],[0 0 1 1-e 0+e 0+e],c2);patch([0 0 1 1-e 0+e 0+e],[0 1 1 1-e 1-e 0+e],c3);plot([0 1 1 0 0],[0 0 1 1 0]);
  wires:
  Input/1 -> Process Input 1/1(x)
  Process Output 1/1(y) -> Output/1
  Process Input 1/1(p) -> Layer 1/1("p{1}")
  Layer 1/1("a{1}") -> [feedback1]
  [feedback1] -> Layer 2/1("a{1} ")
  Layer 2/1("a{2}") -> Process Output 1/1(a)

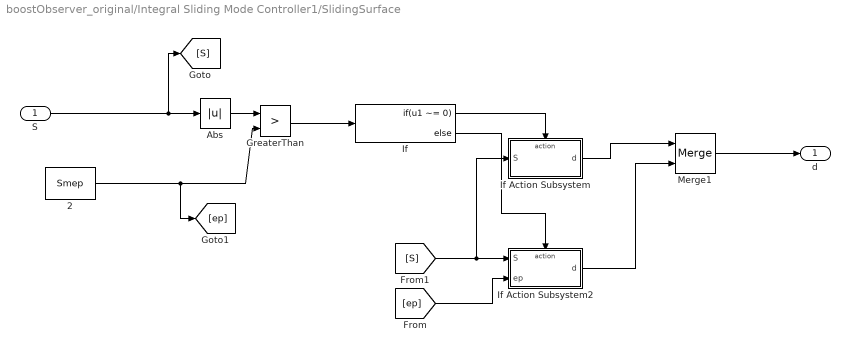
== system boostObserver_original/Integral Sliding Mode Controller1/SlidingSurface ==
  S : Inport
  "    2" : Constant  Value=Smep
  Abs : Abs
  GreaterThan : RelationalOperator  Operator=>  OutDataTypeStr=boolean  RndMeth=Simplest
  If : If  IfExpression=u1 ~= 0
  If Action Subsystem : Subsystem  TreatAsAtomicUnit=on
  If Action Subsystem2 : Subsystem  TreatAsAtomicUnit=on
  Merge1 : Merge
  d : Outport
  wires:
  "    2"/1 -> GreaterThan/2, [ep]
  Merge1/1 -> d/1
  GreaterThan/1 -> If/1
  Abs/1 -> GreaterThan/1
  If Action Subsystem/1(d) -> Merge1/1
  S/1 -> Abs/1, [S]
  [ep] -> If Action Subsystem2/2(ep)
  If/1 -> If Action Subsystem/Action
  If/2 -> If Action Subsystem2/Action
  [S] -> If Action Subsystem2/1(S), If Action Subsystem/1(S)
  If Action Subsystem2/1(d) -> Merge1/2

== system boostObserver_original/Fault Identification/Pattern Recognition Neural Network/Layer 1 ==
  "p{1}" : Inport  PortDimensions=2
      mask Display: e = 0.06;c1 = [120 230 180]/255;c2 = ([120 230 180]+0)/(256+128);c3 = ([120 230 180]+128)/(256+128);patch([0 1 1 0],[0 0 1 1],c1);patch([0 1 1 1-e 1-e 0+e],[0 0 1 1-e 0+e 0+e],c2);patch([0 0 1 1-e 0+e 0+e],[0 1 1 1-e 1-e 0+e],c3);plot([0 1 1 0 0],[0 0 1 1 0]);
  Delays 1 : Subsystem
      mask Display: e = 0.06;c1 = [120 150 230]/255;c2 = ([120 150 230]+0)/383;c3 = ([120 150 230]+128)/383;patch([0 1 1 0],[0 0 1 1],c1);patch([0 1 1 1-e 1-e 0+e],[0 0 1 1-e 0+e 0+e],c2);patch([0 0 1 1-e 0+e 0+e],[0 1 1 1-e 1-e 0+e],c3);plot([0 1 1 0 0],[0 0 1 1 0]);disp('0');
  "IW{1,1}" : Subsystem
      mask Display: e = 0.06;c1 = [120 150 230]/255;c2 = ([120 150 230]+0)/383;c3 = ([120 150 230]+128)/383;patch([0 1 1 0],[0 0 1 1],c1);patch([0 1 1 1-e 1-e 0+e],[0 0 1 1-e 0+e 0+e],c2);patch([0 0 1 1-e 0+e 0+e],[0 1 1 1-e 1-e 0+e],c3);plot([0 1 1 0 0],[0 0 1 1 0]);disp('W');
  "b{1}" : Constant  Value=[1.22077261248049051545194743084721267223358154296875;-0.1998329780659983956336844812540221028029918670654296875;-7.21506241785457103077305873739533126354217529296875;14.0631283131668478603160110651515424251556396484375]
      mask Display: e = 0.06;c1 = [120 150 230]/255;c2 = ([120 150 230]+0)/383;c3 = ([120 150 230]+128)/383;patch([0 1 1 0],[0 0 1 1],c1);patch([0 1 1 1-e 1-e 0+e],[0 0 1 1-e 0+e 0+e],c2);patch([0 0 1 1-e 0+e 0+e],[0 1 1 1-e 1-e 0+e],c3);plot([0 1 1 0 0],[0 0 1 1 0]);disp('b');
  netsum : Sum  Inputs=2  InputSameDT=on  SaturateOnIntegerOverflow=on  OutDataTypeStr=Inherit: Same as first input
      mask Display: e = 0.06;c1 = [120 150 230]/255;c2 = ([120 150 230]+0)/383;c3 = ([120 150 230]+128)/383;patch([0 1 1 0],[0 0 1 1],c1);patch([0 1 1 1-e 1-e 0+e],[0 0 1 1-e 0+e 0+e],c2);patch([0 0 1 1-e 0+e 0+e],[0 1 1 1-e 1-e 0+e],c3);plot([0 1 1 0 0],[0 0 1 1 0]);disp('+');
  tansig : neural/Transfer Functions/tansig
  "a{1}" : Outport  InitialOutput=[0;0;0;0]
      mask Display: e = 0.06;c1 = [120 230 180]/255;c2 = ([120 230 180]+0)/(256+128);c3 = ([120 230 180]+128)/(256+128);patch([0 1 1 0],[0 0 1 1],c1);patch([0 1 1 1-e 1-e 0+e],[0 0 1 1-e 0+e 0+e],c2);patch([0 0 1 1-e 0+e 0+e],[0 1 1 1-e 1-e 0+e],c3);plot([0 1 1 0 0],[0 0 1 1 0]);
  wires:
  "p{1}"/1 -> Delays 1/1("p{1}")
  Delays 1/1("pd{1,1}") -> "IW{1,1}"/1("pd{1,1}")
  "IW{1,1}"/1("iz{1,1}") -> netsum/1
  "b{1}"/1 -> netsum/2
  netsum/1 -> tansig/1
  tansig/1 -> "a{1}"/1

== system boostObserver_original/Fault Identification/Pattern Recognition Neural Network/Layer 2 ==
  "a{1} " : Inport  PortDimensions=4
      mask Display: e = 0.06;c1 = [120 230 180]/255;c2 = ([120 230 180]+0)/(256+128);c3 = ([120 230 180]+128)/(256+128);patch([0 1 1 0],[0 0 1 1],c1);patch([0 1 1 1-e 1-e 0+e],[0 0 1 1-e 0+e 0+e],c2);patch([0 0 1 1-e 0+e 0+e],[0 1 1 1-e 1-e 0+e],c3);plot([0 1 1 0 0],[0 0 1 1 0]);
  Delays 1 : Subsystem
      mask Display: e = 0.06;c1 = [120 150 230]/255;c2 = ([120 150 230]+0)/383;c3 = ([120 150 230]+128)/383;patch([0 1 1 0],[0 0 1 1],c1);patch([0 1 1 1-e 1-e 0+e],[0 0 1 1-e 0+e 0+e],c2);patch([0 0 1 1-e 0+e 0+e],[0 1 1 1-e 1-e 0+e],c3);plot([0 1 1 0 0],[0 0 1 1 0]);disp('0');
  "LW{2,1}" : Subsystem
      mask Display: e = 0.06;c1 = [120 150 230]/255;c2 = ([120 150 230]+0)/383;c3 = ([120 150 230]+128)/383;patch([0 1 1 0],[0 0 1 1],c1);patch([0 1 1 1-e 1-e 0+e],[0 0 1 1-e 0+e 0+e],c2);patch([0 0 1 1-e 0+e 0+e],[0 1 1 1-e 1-e 0+e],c3);plot([0 1 1 0 0],[0 0 1 1 0]);disp('W');
  "b{2}" : Constant  Value=[-0.28327165505055251770727409166283905506134033203125;-0.418393772523750373526496559861698187887668609619140625;0.2351244550115182130323177034370019100606441497802734375;1.90710436787325487983935090596787631511688232421875;-1.3761924879736036064770132725243456661701202392578125]
      mask Display: e = 0.06;c1 = [120 150 230]/255;c2 = ([120 150 230]+0)/383;c3 = ([120 150 230]+128)/383;patch([0 1 1 0],[0 0 1 1],c1);patch([0 1 1 1-e 1-e 0+e],[0 0 1 1-e 0+e 0+e],c2);patch([0 0 1 1-e 0+e 0+e],[0 1 1 1-e 1-e 0+e],c3);plot([0 1 1 0 0],[0 0 1 1 0]);disp('b');
  netsum : Sum  Inputs=2  InputSameDT=on  SaturateOnIntegerOverflow=on  OutDataTypeStr=Inherit: Same as first input
      mask Display: e = 0.06;c1 = [120 150 230]/255;c2 = ([120 150 230]+0)/383;c3 = ([120 150 230]+128)/383;patch([0 1 1 0],[0 0 1 1],c1);patch([0 1 1 1-e 1-e 0+e],[0 0 1 1-e 0+e 0+e],c2);patch([0 0 1 1-e 0+e 0+e],[0 1 1 1-e 1-e 0+e],c3);plot([0 1 1 0 0],[0 0 1 1 0]);disp('+');
  softmax : neural/Transfer Functions/softmax
      settings: SourceProductBaseCode=NN
  "a{2}" : Outport  InitialOutput=[0;0;0;0;0]
      mask Display: e = 0.06;c1 = [120 230 180]/255;c2 = ([120 230 180]+0)/(256+128);c3 = ([120 230 180]+128)/(256+128);patch([0 1 1 0],[0 0 1 1],c1);patch([0 1 1 1-e 1-e 0+e],[0 0 1 1-e 0+e 0+e],c2);patch([0 0 1 1-e 0+e 0+e],[0 1 1 1-e 1-e 0+e],c3);plot([0 1 1 0 0],[0 0 1 1 0]);
  wires:
  "a{1} "/1 -> Delays 1/1("p{2}")
  Delays 1/1("pd{2,1}") -> "LW{2,1}"/1("ad{2,1}")
  "LW{2,1}"/1("lz{2,1}") -> netsum/1
  "b{2}"/1 -> netsum/2
  netsum/1 -> softmax/1
  softmax/1 -> "a{2}"/1

== system boostObserver_original/Fault Identification/Pattern Recognition Neural Network/Process Input 1 ==
  x : Inport  PortDimensions=2
      mask Display: e = 0.06;c1 = [120 230 180]/255;c2 = ([120 230 180]+0)/(256+128);c3 = ([120 230 180]+128)/(256+128);patch([0 1 1 0],[0 0 1 1],c1);patch([0 1 1 1-e 1-e 0+e],[0 0 1 1-e 0+e 0+e],c2);patch([0 0 1 1-e 0+e 0+e],[0 1 1 1-e 1-e 0+e],c3);plot([0 1 1 0 0],[0 0 1 1 0]);
  mapminmax : neural/Processing Functions/mapminmax  xmin=[0;0]  xmax=[11058.6889152982585073914378881;200.235307480860427631341735832]  ymin=-1  ymax=1
  p : Outport  PortDimensions=2
      mask Display: e = 0.06;c1 = [120 230 180]/255;c2 = ([120 230 180]+0)/(256+128);c3 = ([120 230 180]+128)/(256+128);patch([0 1 1 0],[0 0 1 1],c1);patch([0 1 1 1-e 1-e 0+e],[0 0 1 1-e 0+e 0+e],c2);patch([0 0 1 1-e 0+e 0+e],[0 1 1 1-e 1-e 0+e],c3);plot([0 1 1 0 0],[0 0 1 1 0]);
  wires:
  x/1 -> mapminmax/1
  mapminmax/1 -> p/1

== system boostObserver_original/Fault Identification/Pattern Recognition Neural Network/Process Output 1 ==
  a : Inport  PortDimensions=5
      mask Display: e = 0.06;c1 = [120 230 180]/255;c2 = ([120 230 180]+0)/(256+128);c3 = ([120 230 180]+128)/(256+128);patch([0 1 1 0],[0 0 1 1],c1);patch([0 1 1 1-e 1-e 0+e],[0 0 1 1-e 0+e 0+e],c2);patch([0 0 1 1-e 0+e 0+e],[0 1 1 1-e 1-e 0+e],c3);plot([0 1 1 0 0],[0 0 1 1 0]);
  y : Outport  PortDimensions=5
      mask Display: e = 0.06;c1 = [120 230 180]/255;c2 = ([120 230 180]+0)/(256+128);c3 = ([120 230 180]+128)/(256+128);patch([0 1 1 0],[0 0 1 1],c1);patch([0 1 1 1-e 1-e 0+e],[0 0 1 1-e 0+e 0+e],c2);patch([0 0 1 1-e 0+e 0+e],[0 1 1 1-e 1-e 0+e],c3);plot([0 1 1 0 0],[0 0 1 1 0]);
  wires:
  a/1 -> y/1

== system boostObserver_original/Integral Sliding Mode Controller1/SlidingSurface/If Action Subsystem ==
  S : Inport
  Action Port : ActionPort  ActionPortLabel=if(u1 ~= 0)
  Sign : Signum
  d : Outport
  wires:
  Sign/1 -> d/1
  S/1 -> Sign/1

== system boostObserver_original/Integral Sliding Mode Controller1/SlidingSurface/If Action Subsystem2 ==
  S : Inport
  ep : Inport  Port=2
  Action Port : ActionPort  ActionPortLabel=else
  Divide : Product  Inputs=*/
  d : Outport
  wires:
  Divide/1 -> d/1
  ep/1 -> Divide/2
  S/1 -> Divide/1

== system boostObserver_original/Fault Identification/Pattern Recognition Neural Network/Layer 1/Delays 1 ==
  "p{1}" : Inport  PortDimensions=2
      mask Display: e = 0.06;c1 = [120 230 180]/255;c2 = ([120 230 180]+0)/(256+128);c3 = ([120 230 180]+128)/(256+128);patch([0 1 1 0],[0 0 1 1],c1);patch([0 1 1 1-e 1-e 0+e],[0 0 1 1-e 0+e 0+e],c2);patch([0 0 1 1-e 0+e 0+e],[0 1 1 1-e 1-e 0+e],c3);plot([0 1 1 0 0],[0 0 1 1 0]);
  mux : Mux  Inputs=1
      mask Display: e = 0.06;c1 = [120 150 230]/255;c2 = ([120 150 230]+0)/383;c3 = ([120 150 230]+128)/383;patch([0 1 1 0],[0 0 1 1],c1);patch([0 1 1 1-e 1-e 0+e],[0 0 1 1-e 0+e 0+e],c2);patch([0 0 1 1-e 0+e 0+e],[0 1 1 1-e 1-e 0+e],c3);plot([0 1 1 0 0],[0 0 1 1 0]);disp('Mux')
  "pd{1,1}" : Outport
      mask Display: e = 0.06;c1 = [120 230 180]/255;c2 = ([120 230 180]+0)/(256+128);c3 = ([120 230 180]+128)/(256+128);patch([0 1 1 0],[0 0 1 1],c1);patch([0 1 1 1-e 1-e 0+e],[0 0 1 1-e 0+e 0+e],c2);patch([0 0 1 1-e 0+e 0+e],[0 1 1 1-e 1-e 0+e],c3);plot([0 1 1 0 0],[0 0 1 1 0]);
  wires:
  "p{1}"/1 -> mux/1
  mux/1 -> "pd{1,1}"/1
